simulink model "HeartExe_second"  (R2024b)
settings: Solver=ode1  StartTime=0.0  StopTime=30.0  FixedStep=0.5e-3  RelTol=1e-3
model workspace: external: MAT-File N3Data_second.mat (data not in the file)
libraries: Libs_second x151
(part 3 of 3)

== stateflow chart HeartExe_second/cfgs ==
  settings: executeAtInitialization=1
  state Ini
  (default) -> Ini : {Heart=cfgdata_second;}
  data: Heart output; cfgdata_second parameter
